simulink model "WSCC_9bus_static"  (R2018a)
settings: Solver=ode3  StartTime=0.0  StopTime=5  FixedStep=Ts  RelTol=1e-3  EnableMultiTasking=on
InitFcn:
  | Ts=50e-6;
libraries: powerlib x34, powerlib_meascontrol x18
settings Model: Creator=jp536285  LastModifiedBy=acs-mmi
settings DataIOCC: LimitDataPoints=on  SaveFormat=Array
settings OptimizationCC: LifeSpan=inf
settings DebuggingCC: UnderspecifiedInitializationDetection=Classic  MergeDetectMultiDrivingBlocksExec=none  SolverPrmCheckMsg=warning  UnconnectedInputMsg=none  UnconnectedOutputMsg=none  UnconnectedLineMsg=none  StateNameClashWarn=warning  SFUnexpectedBacktrackingDiag=warning  SFNoUnconditionalDefaultTransitionDiag=warning  SFExecutionAtInitializationDiag=none
settings HardwareCC: ProdBitPerPointer=32  ProdBitPerSizeT=32  ProdBitPerPtrDiffT=32  ProdLargestAtomicFloat=None  ProdIntDivRoundTo=Undefined  ProdEndianess=Unspecified  ProdWordSize=32  ProdHWDeviceType=32-bit Generic
settings ModelReferenceCC: PropagateSignalLabelsOutOfModel=off
settings CodeAppCC: StateflowObjectComments=on
settings GRTTargetCC: TargetLangStandard=C89/C90 (ANSI)  GeneratePreprocessorConditionals=Disable all
settings ConfigComp: CovMetricSettings=dw  CovHtmlReporting=on  CovSaveCumulativeToWorkspaceVar=on  CovSaveSingleToWorkspaceVar=on  CovExternalEMLEnable=off  CovSFcnEnable=off
settings SimscapeCC: SimscapeNormalizeSystem=off

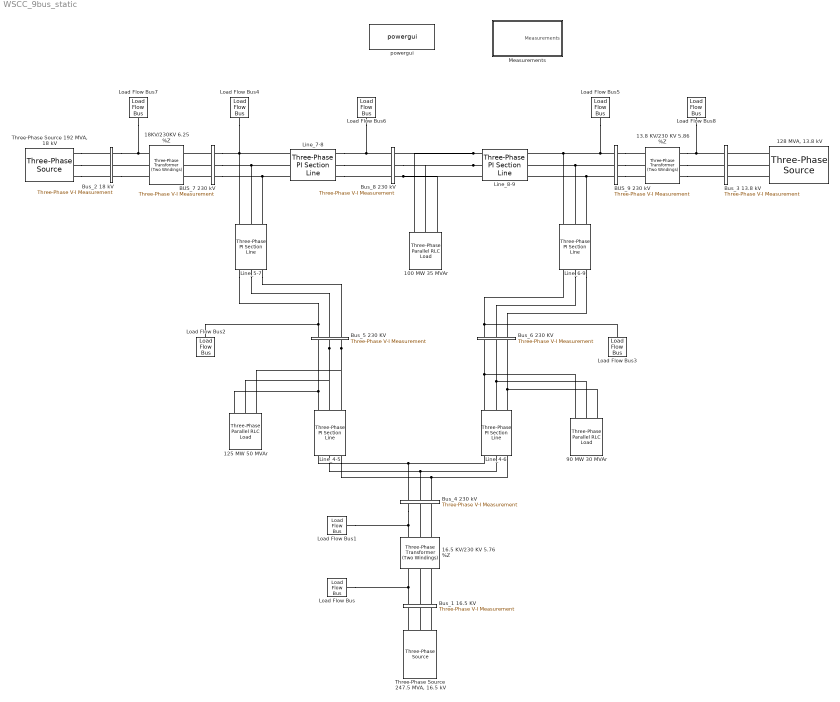
== system WSCC_9bus_static ==
  100 MW 35 MVAr : powerlib/Elements/Three-Phase Parallel RLC Load  LConnTagsString=A|B|C  Configuration=Y (grounded)  NominalVoltage=(230000)*1.01602  Vabc=[1e3 1e3 1e3]  Vabcp=[1e3 1e3 1e3]  NominalFrequency=60  UnbalancedPower=off  ActivePower=100e6  InductivePower=35e6  CapacitivePower=0  Pabc=[10e3 9e3 11e3]  QLabc=[100 90 110]  QCabc=[100 90 110]  Pabcp=[10e3 9e3 11e3]  QLabcp=[100 90 110]  QCabcp=[100 90 110]  Measurements=None  LoadType=constant PQ
  125 MW 50 MVAr : powerlib/Elements/Three-Phase Parallel RLC Load  LConnTagsString=A|B|C  Configuration=Y (grounded)  NominalVoltage=(230000)*0.996139  Vabc=[1e3 1e3 1e3]  Vabcp=[1e3 1e3 1e3]  NominalFrequency=60  UnbalancedPower=off  ActivePower=125e6  InductivePower=50e6  CapacitivePower=0  Pabc=[10e3 9e3 11e3]  QLabc=[100 90 110]  QCabc=[100 90 110]  Pabcp=[10e3 9e3 11e3]  QLabcp=[100 90 110]  QCabcp=[100 90 110]  Measurements=None  LoadType=constant PQ
  "128 MVA, 13.8 kV" : powerlib/Electrical Sources/Three-Phase Source  InternalConnection=Yg  VoltagePhases=off  Voltage=(13800)*1.025  PhaseAngle=4.6126  Voltage_phases=[25e3 25e3 25e3]/sqrt(3)  PhaseAngles_phases=[0 -120 +120]  Frequency=60  NonIdealSource=off  SpecifyImpedance=on  Resistance=0.529  Inductance=0.0140  ShortCircuitLevel=128e6  BaseVoltage=13.8e3  XRratio=100000  BusType=PV  Pref=85000000  Qref=0  Prefabc=[10e3, 10e3, 10e3]  Qrefabc=[0, 0, 0]  Qmin=-inf  Qmax=inf
  13.8 KV/230 KV 5.86 %Z : powerlib/Elements/Three-Phase Transformer (Two Windings)  Winding1Connection=Yg  Winding2Connection=Yg  CoreType=Three single-phase transformers  SetSaturation=off  Hysteresis=off  DataFile='hysteresis'  SetInitialFlux=off  Measurements=None  UNITS=SI  NominalPower=[ 100e6 60 ]  Winding1=[13800 0 0]  Winding2=[230e3 1e-06 0.0822 ]  Rm=Inf  Lm=Inf  L0=0.5  Saturation=[0 0;14.2 35.866;5916.6 45.43]  InitialFluxes=[23.911 -23.911 20.922]  MoreParameters=off  BreakLoop=off  DataType=on  TransfoNumber=1
  "16.5 KV/230 KV 5.76 %Z     " : powerlib/Elements/Three-Phase Transformer (Two Windings)  Winding1Connection=Yg  Winding2Connection=Yg  CoreType=Three single-phase transformers  SetSaturation=off  Hysteresis=off  DataFile='hysteresis'  SetInitialFlux=off  Measurements=None  UNITS=SI  NominalPower=[ 100e6 60 ]  Winding1=[16500 0 0]  Winding2=[230e3 1e-6 0.0808 ]  Rm=Inf  Lm=Inf  L0=0.5  Saturation=[0 0;29.394 42.883;12247 54.319]  InitialFluxes=[28.589 -28.589 25.015]  MoreParameters=off  BreakLoop=off  DataType=on  TransfoNumber=1
  18KV/230KV 6.25 %Z : powerlib/Elements/Three-Phase Transformer (Two Windings)  Winding1Connection=Yg  Winding2Connection=Yg  CoreType=Three single-phase transformers  SetSaturation=off  Hysteresis=off  DataFile='hysteresis'  SetInitialFlux=off  Measurements=None  UNITS=SI  NominalPower=[ 100e6 60 ]  Winding1=[18000 0 0]  Winding2=[230e3 1e-6 0.0877]  Rm=Inf  Lm=Inf  L0=0.5  Saturation=[0 0;10.887 46.782;4536.1 59.257]  InitialFluxes=[31.188 -31.188 27.289]  MoreParameters=off  BreakLoop=off  DataType=on  TransfoNumber=1
  90 MW 30 MVAr : powerlib/Elements/Three-Phase Parallel RLC Load  LConnTagsString=A|B|C  Configuration=Y (grounded)  NominalVoltage=(230000)*1.01311  Vabc=[1e3 1e3 1e3]  Vabcp=[1e3 1e3 1e3]  NominalFrequency=60  UnbalancedPower=off  ActivePower=90e6  InductivePower=30e6  CapacitivePower=0  Pabc=[10e3 9e3 11e3]  QLabc=[100 90 110]  QCabc=[100 90 110]  Pabcp=[10e3 9e3 11e3]  QLabcp=[100 90 110]  QCabcp=[100 90 110]  Measurements=None  LoadType=constant PQ
  BUS_7 230 kV : powerlib/Measurements/Three-Phase V-I Measurement  VoltageMeasurement=phase-to-phase  SetLabelV=on  LabelV=Vabc_7  Vpu=off  VpuLL=off  CurrentMeasurement=yes  SetLabelI=on  LabelI=Iabc_7  Ipu=off  Pbase=100e6  Vbase=230e3  OutputType=Complex  PhasorSimulation=off  PSBequivalent=0
  BUS_9 230 kV : powerlib/Measurements/Three-Phase V-I Measurement  VoltageMeasurement=phase-to-phase  SetLabelV=on  LabelV=Vabc_9  Vpu=off  VpuLL=off  CurrentMeasurement=yes  SetLabelI=on  LabelI=Iabc_9  Ipu=off  Pbase=100e6  Vbase=230e3  OutputType=Complex  PhasorSimulation=off  PSBequivalent=0
  Bus_1 16.5 KV : powerlib/Measurements/Three-Phase V-I Measurement  VoltageMeasurement=phase-to-phase  SetLabelV=on  LabelV=Vabc_1  Vpu=off  VpuLL=off  CurrentMeasurement=yes  SetLabelI=on  LabelI=Iabc_1  Ipu=off  Pbase=100e6  Vbase=16.5e3  OutputType=Complex  PhasorSimulation=off  PSBequivalent=0
  Bus_2 18 kV : powerlib/Measurements/Three-Phase V-I Measurement  VoltageMeasurement=phase-to-phase  SetLabelV=on  LabelV=Vabc_2  Vpu=off  VpuLL=off  CurrentMeasurement=yes  SetLabelI=on  LabelI=Iabc_2  Ipu=off  Pbase=100e6  Vbase=18e3  OutputType=Complex  PhasorSimulation=off  PSBequivalent=0
  Bus_3 13.8 kV : powerlib/Measurements/Three-Phase V-I Measurement  VoltageMeasurement=phase-to-phase  SetLabelV=on  LabelV=Vabc_3  Vpu=off  VpuLL=off  CurrentMeasurement=yes  SetLabelI=on  LabelI=Iabc_3  Ipu=off  Pbase=100e6  Vbase=13.8e3  OutputType=Complex  PhasorSimulation=off  PSBequivalent=0
  Bus_4 230 kV : powerlib/Measurements/Three-Phase V-I Measurement  VoltageMeasurement=phase-to-phase  SetLabelV=on  LabelV=Vabc_4  Vpu=off  VpuLL=off  CurrentMeasurement=yes  SetLabelI=on  LabelI=Iabc_4  Ipu=off  Pbase=100e6  Vbase=230e3  OutputType=Complex  PhasorSimulation=off  PSBequivalent=0
  Bus_5 230 KV : powerlib/Measurements/Three-Phase V-I Measurement  VoltageMeasurement=phase-to-phase  SetLabelV=on  LabelV=Vabc_5  Vpu=off  VpuLL=off  CurrentMeasurement=yes  SetLabelI=on  LabelI=Iabc_5  Ipu=off  Pbase=100e6  Vbase=230e3  OutputType=Complex  PhasorSimulation=off  PSBequivalent=0
  Bus_6 230 KV : powerlib/Measurements/Three-Phase V-I Measurement  VoltageMeasurement=phase-to-phase  SetLabelV=on  LabelV=Vabc_6  Vpu=off  VpuLL=off  CurrentMeasurement=yes  SetLabelI=on  LabelI=Iabc_6  Ipu=off  Pbase=100e6  Vbase=230e3  OutputType=Complex  PhasorSimulation=off  PSBequivalent=0
  Bus_8 230 kV : powerlib/Measurements/Three-Phase V-I Measurement  VoltageMeasurement=phase-to-phase  SetLabelV=on  LabelV=Vabc_8  Vpu=off  VpuLL=off  CurrentMeasurement=yes  SetLabelI=on  LabelI=Iabc_8  Ipu=off  Pbase=100e6  Vbase=230e3  OutputType=Complex  PhasorSimulation=off  PSBequivalent=0
  Line_4-5 : powerlib/Elements/Three-Phase PI Section Line  LConnTagsString=a|b|c  RConnTagsString=A|B|C  Frequency=60  Resistances=[ 05.29 15.87 ]  Inductances="[ 0.1192  0.3578 ]"  Capacitances=[0.8825e-6 0.8825e-6 ]  Length=1
      settings: SourceProductName=Simscape Power Systems
  Line_4-6 : powerlib/Elements/Three-Phase PI Section Line  LConnTagsString=a|b|c  RConnTagsString=A|B|C  Frequency=60  Resistances=[ 8.993 26.979]  Inductances="[ 0.1291  0.3873 ]"  Capacitances=[ 0.7922e-6 0.7922e-6 ]  Length=1
      settings: SourceProductName=Simscape Power Systems
  Line_5-7 : powerlib/Elements/Three-Phase PI Section Line  LConnTagsString=a|b|c  RConnTagsString=A|B|C  Frequency=60  Resistances=[ 16.928 50.784 ]  Inductances="[ 0.2259  0.6778 ]"  Capacitances=[1.5343e-6 1.5343e-6]  Length=1
      settings: SourceProductName=Simscape Power Systems
  Line_6-9 : powerlib/Elements/Three-Phase PI Section Line  LConnTagsString=a|b|c  RConnTagsString=A|B|C  Frequency=60  Resistances=[ 20.631 61.893]  Inductances="[ 0.2385  0.7156 ]"  Capacitances=[1.7951e-6 1.7951e-6 ]  Length=1
      settings: SourceProductName=Simscape Power Systems
  Line_7-8 : powerlib/Elements/Three-Phase PI Section Line  LConnTagsString=a|b|c  RConnTagsString=A|B|C  Frequency=60  Resistances=[ 4.4965 13.4895 ]  Inductances="[ 0.101  0.3031 ]"  Capacitances=[0.7471e-6 0.7471e-6]  Length=1
      settings: SourceProductName=Simscape Power Systems
  Line_8-9 : powerlib/Elements/Three-Phase PI Section Line  LConnTagsString=a|b|c  RConnTagsString=A|B|C  Frequency=60  Resistances=[ 6.2951 18.8853 ]  Inductances="[ 0.1414  0.4243 ]"  Capacitances=[1.047995e-6 1.047995e-6 ]  Length=1
      settings: SourceProductName=Simscape Power Systems
  Load Flow Bus : powerlib/Measurements/Load Flow Bus  LConnTagsString=a  Phases=single  Connectors=on one side  ID=BUS_1  Vbase=16.5e3  Vref=1.04  Vangle=0  VLF=1.04  VLFb=1  VLFc=1  angleLF=0  angleLFb=0  angleLFc=0
      settings: AttributesFormatString=%<ID>\n%<Vbase>V\n%<VLF>pu\n%<angleLF>deg.  SourceProductName=Simscape Power Systems
  Load Flow Bus1 : powerlib/Measurements/Load Flow Bus  LConnTagsString=a  Phases=single  Connectors=on one side  ID=BUS_4  Vbase=230e3  Vref=1  Vangle=0  VLF=1.026  VLFb=1  VLFc=1  angleLF=-2.213  angleLFb=0  angleLFc=0
      settings: AttributesFormatString=%<ID>\n%<Vbase>V\n%<VLF>pu\n%<angleLF>deg.  SourceProductName=Simscape Power Systems
  Load Flow Bus2 : powerlib/Measurements/Load Flow Bus  LConnTagsString=a  Phases=single  Connectors=on one side  ID=BUS_5  Vbase=230e3  Vref=1  Vangle=0  VLF=0.9961  VLFb=1  VLFc=1  angleLF=-3.978  angleLFb=0  angleLFc=0
      settings: AttributesFormatString=%<ID>\n%<Vbase>V\n%<VLF>pu\n%<angleLF>deg.  SourceProductName=Simscape Power Systems
  Load Flow Bus3 : powerlib/Measurements/Load Flow Bus  LConnTagsString=a  Phases=single  Connectors=on one side  ID=BUS_6  Vbase=230e3  Vref=1  Vangle=0  VLF=1.013  VLFb=1  VLFc=1  angleLF=-3.68  angleLFb=0  angleLFc=0
      settings: AttributesFormatString=%<ID>\n%<Vbase>V\n%<VLF>pu\n%<angleLF>deg.  SourceProductName=Simscape Power Systems
  Load Flow Bus4 : powerlib/Measurements/Load Flow Bus  LConnTagsString=a  Phases=single  Connectors=on one side  ID=BUS_7  Vbase=230e3  Vref=1  Vangle=0  VLF=1.026  VLFb=1  VLFc=1  angleLF=3.666  angleLFb=0  angleLFc=0
      settings: AttributesFormatString=%<ID>\n%<Vbase>V\n%<VLF>pu\n%<angleLF>deg.  SourceProductName=Simscape Power Systems
  Load Flow Bus5 : powerlib/Measurements/Load Flow Bus  LConnTagsString=a  Phases=single  Connectors=on one side  ID=BUS_9  Vbase=230e3  Vref=1  Vangle=0  VLF=1.032  VLFb=1  VLFc=1  angleLF=1.916  angleLFb=0  angleLFc=0
      settings: AttributesFormatString=%<ID>\n%<Vbase>V\n%<VLF>pu\n%<angleLF>deg.  SourceProductName=Simscape Power Systems
  Load Flow Bus6 : powerlib/Measurements/Load Flow Bus  LConnTagsString=a  Phases=single  Connectors=on one side  ID=BUS_8  Vbase=230e3  Vref=1  Vangle=0  VLF=1.016  VLFb=1  VLFc=1  angleLF=0.681  angleLFb=0  angleLFc=0
      settings: AttributesFormatString=%<ID>\n%<Vbase>V\n%<VLF>pu\n%<angleLF>deg.  SourceProductName=Simscape Power Systems
  Load Flow Bus7 : powerlib/Measurements/Load Flow Bus  LConnTagsString=a  Phases=single  Connectors=on one side  ID=BUS_2  Vbase=18e3  Vref=1.025  Vangle=0  VLF=1.025  VLFb=1  VLFc=1  angleLF=9.226  angleLFb=0  angleLFc=0
      settings: AttributesFormatString=%<ID>\n%<Vbase>V\n%<VLF>pu\n%<angleLF>deg.  SourceProductName=Simscape Power Systems
  Load Flow Bus8 : powerlib/Measurements/Load Flow Bus  LConnTagsString=a  Phases=single  Connectors=on one side  ID=BUS_3  Vbase=13.8e3  Vref=1.025  Vangle=0  VLF=1.025  VLFb=1  VLFc=1  angleLF=4.613  angleLFb=0  angleLFc=0
      settings: AttributesFormatString=%<ID>\n%<Vbase>V\n%<VLF>pu\n%<angleLF>deg.  SourceProductName=Simscape Power Systems
  Measurements : Subsystem
  "Three-Phase Source 192 MVA, 18 kV" : powerlib/Electrical Sources/Three-Phase Source  InternalConnection=Yg  VoltagePhases=off  Voltage=(18000)*1.025  PhaseAngle=9.2261  Voltage_phases=[25e3 25e3 25e3]/sqrt(3)  PhaseAngles_phases=[0 -120 +120]  Frequency=60  NonIdealSource=off  SpecifyImpedance=on  Resistance=0.8929  Inductance=16.58e-3  ShortCircuitLevel=192e6  BaseVoltage=18e3  XRratio=100000  BusType=PV  Pref=163e6  Qref=0  Prefabc=[10e3, 10e3, 10e3]  Qrefabc=[0, 0, 0]  Qmin=-inf  Qmax=inf
  "Three-Phase Source 247.5 MVA, 16.5 kV" : powerlib/Electrical Sources/Three-Phase Source  InternalConnection=Yg  VoltagePhases=off  Voltage=(16500)*1.04  PhaseAngle=0  Voltage_phases=[25e3 25e3 25e3]/sqrt(3)  PhaseAngles_phases=[0 -120 +120]  Frequency=60  NonIdealSource=off  SpecifyImpedance=on  Resistance=0.8929  Inductance=16.58e-3  ShortCircuitLevel=247.5e6  BaseVoltage=16.5e3  XRratio=100000  BusType=swing  Pref=10e3  Qref=0  Prefabc=[10e3, 10e3, 10e3]  Qrefabc=[0, 0, 0]  Qmin=-inf  Qmax=inf
  powergui : powerlib/powergui  Priority=1  SimulationMode=Discrete  SampleTime=Ts  frequency=60  Iterations=50  frequencyindice=60  Pbase=10e7  ErrMax=1e-05  UnitsV=kV  UnitsW=MW  buscounter=0  FunctionMessages=off  echomessages=off  EnableUseOfTLC=off  CurrentSourceSwitches=off  DisableSnubberDevices=off  DisableRonSwitches=off  DisableVfSwitches=off  DisplayEquations=off  SolverType=Backward Euler  Interpol=on  ExternalGateDelay=off  methode=off  Ts=0  x0status=blocks  SPID=on  SwTol=0  HookPort=off  RestoreLinks=warning  ResistiveCurrentMeasurement=off  Frange=[0:2:500]  Ylog=off  Xlog=on  ShowGrid=off  save=off  variable=ZData  structure=0  ZoomFFT=off  StartTime=0.0  cycles=1  DisplayStyle=1  fundamental=60  FreqAxis=off  MaxFrequency=1000  frequencyindicesteady=1  RmsSteady=1  display=off
  connections:
  "Three-Phase Source 192 MVA, 18 kV"/RConn2 -- Bus_2 18 kV/LConn2
  18KV/230KV 6.25 %Z/LConn2 -- Bus_2 18 kV/RConn2
  Bus_2 18 kV/RConn1 -- Load Flow Bus7/LConn1 -- 18KV/230KV 6.25 %Z/LConn1
  Bus_2 18 kV/RConn3 -- 18KV/230KV 6.25 %Z/LConn3
  Load Flow Bus8/LConn1 -- 13.8 KV/230 KV 5.86 %Z/LConn1 -- Bus_3 13.8 kV/LConn1
  13.8 KV/230 KV 5.86 %Z/LConn2 -- Bus_3 13.8 kV/LConn2
  13.8 KV/230 KV 5.86 %Z/LConn3 -- Bus_3 13.8 kV/LConn3
  "Three-Phase Source 247.5 MVA, 16.5 kV"/RConn1 -- Bus_1 16.5 KV/RConn1
  "Three-Phase Source 247.5 MVA, 16.5 kV"/RConn2 -- Bus_1 16.5 KV/RConn2
  "Three-Phase Source 247.5 MVA, 16.5 kV"/RConn3 -- Bus_1 16.5 KV/RConn3
  Bus_1 16.5 KV/LConn1 -- Load Flow Bus/LConn1 -- "16.5 KV/230 KV 5.76 %Z     "/LConn1
  Bus_1 16.5 KV/LConn3 -- "16.5 KV/230 KV 5.76 %Z     "/LConn3
  Bus_1 16.5 KV/LConn2 -- "16.5 KV/230 KV 5.76 %Z     "/LConn2
  Load Flow Bus1/LConn1 -- Bus_4 230 kV/RConn1 -- "16.5 KV/230 KV 5.76 %Z     "/RConn1
  "16.5 KV/230 KV 5.76 %Z     "/RConn2 -- Bus_4 230 kV/RConn2
  Line_8-9/LConn1 -- 100 MW 35 MVAr/LConn1 -- Bus_8 230 kV/LConn1
  Line_8-9/LConn2 -- 100 MW 35 MVAr/LConn2 -- Bus_8 230 kV/LConn2
  Bus_8 230 kV/LConn3 -- 100 MW 35 MVAr/LConn3 -- Line_8-9/LConn3
  "16.5 KV/230 KV 5.76 %Z     "/RConn3 -- Bus_4 230 kV/RConn3
  Line_4-5/RConn1 -- 125 MW 50 MVAr/LConn1 -- Bus_5 230 KV/RConn1
  Bus_5 230 KV/RConn2 -- 125 MW 50 MVAr/LConn2 -- Line_4-5/RConn2
  Bus_5 230 KV/RConn3 -- 125 MW 50 MVAr/LConn3 -- Line_4-5/RConn3
  Line_4-6/RConn1 -- 90 MW 30 MVAr/LConn1 -- Bus_6 230 KV/RConn1
  Line_4-6/RConn2 -- 90 MW 30 MVAr/LConn2 -- Bus_6 230 KV/RConn2
  Line_4-6/RConn3 -- 90 MW 30 MVAr/LConn3 -- Bus_6 230 KV/RConn3
  Bus_8 230 kV/RConn1 -- Line_7-8/RConn1 -- Load Flow Bus6/LConn1
  Line_7-8/RConn2 -- Bus_8 230 kV/RConn2
  Line_7-8/RConn3 -- Bus_8 230 kV/RConn3
  Line_5-7/LConn1 -- Load Flow Bus2/LConn1 -- Bus_5 230 KV/LConn1
  Line_5-7/LConn2 -- Bus_5 230 KV/LConn2
  Line_5-7/LConn3 -- Bus_5 230 KV/LConn3
  Bus_6 230 KV/LConn1 -- Load Flow Bus3/LConn1 -- Line_6-9/LConn1
  Line_6-9/LConn2 -- Bus_6 230 KV/LConn2
  Line_6-9/LConn3 -- Bus_6 230 KV/LConn3
  "128 MVA, 13.8 kV"/RConn1 -- Bus_3 13.8 kV/RConn1
  "128 MVA, 13.8 kV"/RConn2 -- Bus_3 13.8 kV/RConn2
  "128 MVA, 13.8 kV"/RConn3 -- Bus_3 13.8 kV/RConn3
  "Three-Phase Source 192 MVA, 18 kV"/RConn3 -- Bus_2 18 kV/LConn3
  "Three-Phase Source 192 MVA, 18 kV"/RConn1 -- Bus_2 18 kV/LConn1
  BUS_7 230 kV/LConn1 -- 18KV/230KV 6.25 %Z/RConn1
  BUS_7 230 kV/LConn2 -- 18KV/230KV 6.25 %Z/RConn2
  BUS_7 230 kV/LConn3 -- 18KV/230KV 6.25 %Z/RConn3
  BUS_7 230 kV/RConn1 -- Load Flow Bus4/LConn1 -- Line_5-7/RConn1 -- Line_7-8/LConn1
  BUS_7 230 kV/RConn2 -- Line_5-7/RConn2 -- Line_7-8/LConn2
  BUS_7 230 kV/RConn3 -- Line_5-7/RConn3 -- Line_7-8/LConn3
  BUS_9 230 kV/RConn1 -- 13.8 KV/230 KV 5.86 %Z/RConn1
  BUS_9 230 kV/RConn2 -- 13.8 KV/230 KV 5.86 %Z/RConn2
  BUS_9 230 kV/RConn3 -- 13.8 KV/230 KV 5.86 %Z/RConn3
  BUS_9 230 kV/LConn1 -- Line_6-9/RConn1 -- Line_8-9/RConn1 -- Load Flow Bus5/LConn1
  BUS_9 230 kV/LConn2 -- Line_6-9/RConn2 -- Line_8-9/RConn2
  BUS_9 230 kV/LConn3 -- Line_6-9/RConn3 -- Line_8-9/RConn3
  Line_4-5/LConn1 -- Bus_4 230 kV/LConn1 -- Line_4-6/LConn1
  Line_4-5/LConn2 -- Bus_4 230 kV/LConn2 -- Line_4-6/LConn2
  Line_4-5/LConn3 -- Bus_4 230 kV/LConn3 -- Line_4-6/LConn3

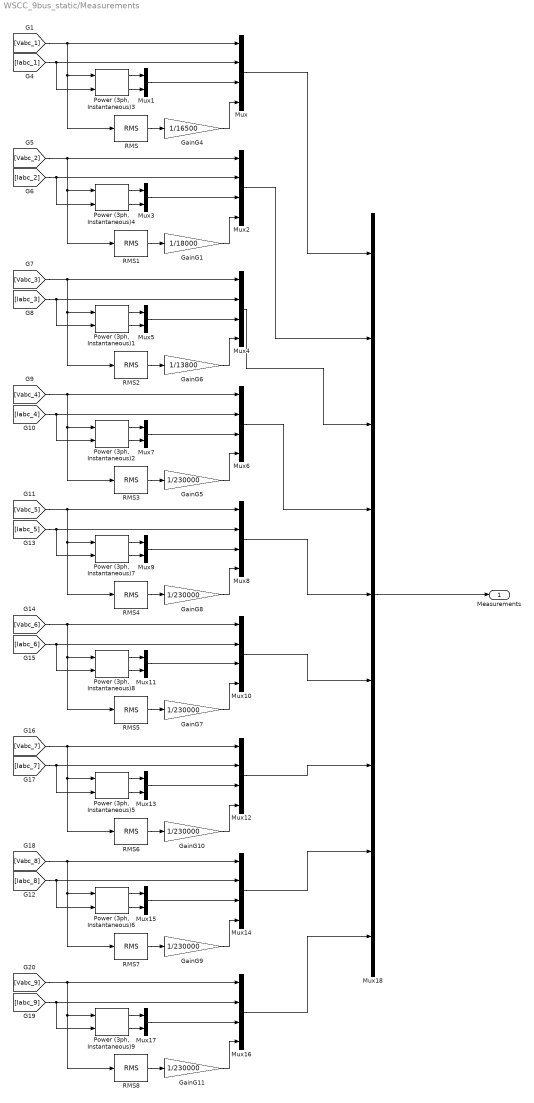
== system WSCC_9bus_static/Measurements ==
  GainG1 : Gain  Gain=1/18000
  GainG{5,7..11} (6 alike) : Gain  Gain=1/230000
  GainG4 : Gain  Gain=1/16500
  GainG6 : Gain  Gain=1/13800
  Mux{,2,4,6,8,10,12,14,16} (9 alike) : Mux
  Mux{1,3,5,7,9,11,13,15,17} (9 alike) : Mux  Inputs=2
  Mux18 : Mux  Inputs=9
  Power (3ph, Instantaneous){1..9} (9 alike) : powerlib_meascontrol/Measurements/Power (3ph, Instantaneous)
      settings: SourceProductName=Simscape Power Systems
  RMS{,1..8} (9 alike) : powerlib_meascontrol/Measurements/RMS  TrueRMS=on  Freq=60  RMSInit=230  Ts=0
  Measurements : Outport
  wires:
  [Vabc_1] -> RMS/1, "Power (3ph, Instantaneous)3"/1, Mux/1
  RMS/1 -> GainG4/1
  [Iabc_1] -> "Power (3ph, Instantaneous)3"/2, Mux/2
  GainG4/1 -> Mux/4
  "Power (3ph, Instantaneous)3"/1 -> Mux1/1
  "Power (3ph, Instantaneous)3"/2 -> Mux1/2
  Mux1/1 -> Mux/3
  "Power (3ph, Instantaneous)4"/2 -> Mux3/2
  [Vabc_2] -> RMS1/1, "Power (3ph, Instantaneous)4"/1, Mux2/1
  [Iabc_2] -> "Power (3ph, Instantaneous)4"/2, Mux2/2
  "Power (3ph, Instantaneous)4"/1 -> Mux3/1
  RMS1/1 -> GainG1/1
  GainG1/1 -> Mux2/4
  Mux3/1 -> Mux2/3
  "Power (3ph, Instantaneous)1"/2 -> Mux5/2
  "Power (3ph, Instantaneous)2"/1 -> Mux7/1
  GainG5/1 -> Mux6/4
  [Iabc_4] -> "Power (3ph, Instantaneous)2"/2, Mux6/2
  RMS3/1 -> GainG5/1
  [Vabc_3] -> RMS2/1, "Power (3ph, Instantaneous)1"/1, Mux4/1
  [Vabc_4] -> RMS3/1, "Power (3ph, Instantaneous)2"/1, Mux6/1
  [Iabc_3] -> "Power (3ph, Instantaneous)1"/2, Mux4/2
  Mux7/1 -> Mux6/3
  "Power (3ph, Instantaneous)1"/1 -> Mux5/1
  RMS2/1 -> GainG6/1
  GainG6/1 -> Mux4/4
  Mux5/1 -> Mux4/3
  "Power (3ph, Instantaneous)2"/2 -> Mux7/2
  "Power (3ph, Instantaneous)7"/2 -> Mux9/2
  "Power (3ph, Instantaneous)8"/1 -> Mux11/1
  GainG7/1 -> Mux10/4
  [Iabc_6] -> "Power (3ph, Instantaneous)8"/2, Mux10/2
  RMS5/1 -> GainG7/1
  [Vabc_5] -> RMS4/1, "Power (3ph, Instantaneous)7"/1, Mux8/1
  [Vabc_6] -> RMS5/1, "Power (3ph, Instantaneous)8"/1, Mux10/1
  [Iabc_5] -> "Power (3ph, Instantaneous)7"/2, Mux8/2
  Mux11/1 -> Mux10/3
  "Power (3ph, Instantaneous)6"/2 -> Mux15/2
  Mux13/1 -> Mux12/3
  RMS6/1 -> GainG10/1
  GainG10/1 -> Mux12/4
  "Power (3ph, Instantaneous)5"/1 -> Mux13/1
  [Vabc_8] -> RMS7/1, "Power (3ph, Instantaneous)6"/1, Mux14/1
  [Iabc_7] -> "Power (3ph, Instantaneous)5"/2, Mux12/2
  [Vabc_7] -> RMS6/1, "Power (3ph, Instantaneous)5"/1, Mux12/1
  Mux15/1 -> Mux14/3
  "Power (3ph, Instantaneous)7"/1 -> Mux9/1
  [Iabc_8] -> "Power (3ph, Instantaneous)6"/2, Mux14/2
  RMS7/1 -> GainG9/1
  "Power (3ph, Instantaneous)6"/1 -> Mux15/1
  RMS4/1 -> GainG8/1
  "Power (3ph, Instantaneous)5"/2 -> Mux13/2
  GainG9/1 -> Mux14/4
  GainG8/1 -> Mux8/4
  Mux9/1 -> Mux8/3
  "Power (3ph, Instantaneous)8"/2 -> Mux11/2
  "Power (3ph, Instantaneous)9"/1 -> Mux17/1
  RMS8/1 -> GainG11/1
  [Iabc_9] -> "Power (3ph, Instantaneous)9"/2, Mux16/2
  "Power (3ph, Instantaneous)9"/2 -> Mux17/2
  GainG11/1 -> Mux16/4
  Mux17/1 -> Mux16/3
  [Vabc_9] -> RMS8/1, "Power (3ph, Instantaneous)9"/1, Mux16/1
  Mux/1 -> Mux18/1
  Mux2/1 -> Mux18/2
  Mux4/1 -> Mux18/3
  Mux6/1 -> Mux18/4
  Mux8/1 -> Mux18/5
  Mux10/1 -> Mux18/6
  Mux12/1 -> Mux18/7
  Mux14/1 -> Mux18/8
  Mux16/1 -> Mux18/9
  Mux18/1 -> Measurements/1
